simulink model "pendulo_simples"  (R2018b)
settings: Solver=VariableStepAuto  StartTime=0.0  StopTime=30.0  RelTol=1e-3
values from neighbouring files (symbols this model uses):
  G = Gp*C2    [LGR_3D.m]    (also in atividade5pts.m = tf(numG, denG); atraso.m = tf(k,den,'IODelay',d); modelo_chan.m = 0.0564; rlocus_pendulo.m = tf(k*1.4^2, [1, 2*1.4*0.19, 1.4^2]))
settings Model: Creator=bernardo  LastModifiedBy=bernardo

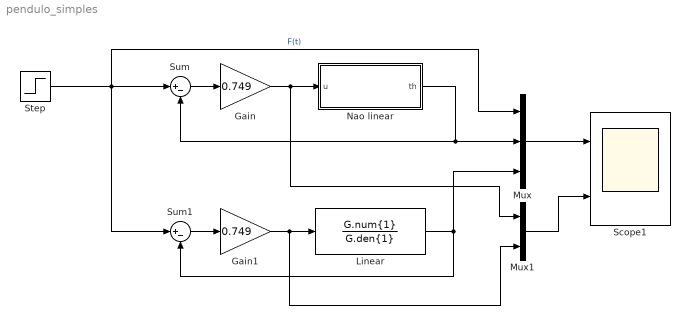
== system pendulo_simples ==
  Gain : Gain  Gain=0.749
  Gain1 : Gain  Gain=0.749
  Linear : TransferFcn  Numerator=G.num{1}  Denominator=G.den{1}
  Mux : Mux  Inputs=3
  Mux1 : Mux  Inputs=2
  Nao linear : Subsystem
  Scope1 : Scope  NumInputPorts=2
  Step : Step  Time=0  SampleTime=0.001
  Sum : Sum  Inputs=|+-
  Sum1 : Sum  Inputs=|+-
  wires:
  Step/1 -> Mux/1, Sum/1, Sum1/1  "F(t)"
  Gain/1 -> Mux1/1, Nao linear/1(u)
  Sum/1 -> Gain/1
  Gain1/1 -> Linear/1, Mux1/2
  Sum1/1 -> Gain1/1
  Linear/1 -> Mux/3, Sum1/2
  Mux/1 -> Scope1/1
  Mux1/1 -> Scope1/2
  Nao linear/1(th) -> Sum/2, Mux/2

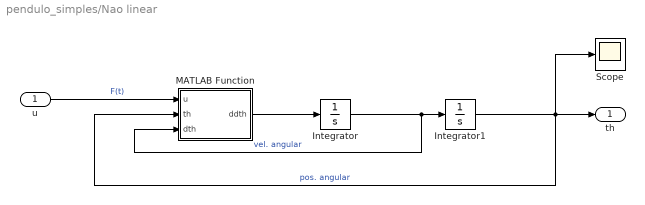
== system pendulo_simples/Nao linear ==
  u : Inport
  Integrator : Integrator
  Integrator1 : Integrator
  MATLAB Function : MATLAB Function  TreatAsAtomicUnit=on
  Scope : Scope
  th : Outport
  wires:
  Integrator/1 -> MATLAB Function/3(dth), Integrator1/1  "vel. angular"
  Integrator1/1 -> Scope/1, th/1, MATLAB Function/2(th)  "pos. angular"
  u/1 -> MATLAB Function/1(u)  "F(t)"
  MATLAB Function/1(ddth) -> Integrator/1

== matlab function pendulo_simples/Nao linear/MATLAB Function ==
  data: u input; ddth output; th input; dth input
function ddth = fcn(u,th,dth)
    m = 0.2;
    L = 0.5;
    g = 9.8;
    k = 1;
    ddth = u/cos(th) + dth*(dth*tan(th) - L*k/cos(th)) - m*g*tan(th);
y = u;
